simulink model "online_hardware_backstepping_controller"  (R2020b)
settings: Solver=FixedStepAuto  StartTime=0.0  StopTime=120  FixedStep=0.01  RelTol=1e-3  EnableMultiTasking=on
libraries: simulink x4, arduinolib x4, arduinosensorlib x1
settings Model: SILPILModeSetting=veronly  ExtModeTrigDuration=2  Creator=Boreth  LastModifiedBy=ONLY-GOD
settings OptimizationCC: EnhancedBackFolding=on  PassReuseOutputArgsAs=Individual arguments  MaxStackSize=64  OptimizeBlockOrder=speed  DifferentSizesBufferReuse=on  EfficientTunableParamExpr=on
settings DebuggingCC: InheritedTsInSrcMsg=none  ParameterTunabilityLossMsg=error  ArithmeticOperatorsInVariantConditions=warning
settings HardwareCC: ProdBitPerPointer=32  ProdBitPerSizeT=32  ProdBitPerPtrDiffT=32  ProdLargestAtomicInteger=Long  ProdLargestAtomicFloat=Double  ProdWordSize=32  ProdHWDeviceType=ARM Compatible->ARM Cortex
settings SFSimCC: MATLABDynamicMemAlloc=off  CustomCodeUndefinedFunction=UseInterfaceOnly
settings RTWCC: Description=Embedded Coder  SystemTargetFile=ert.tlc  HardwareBoard=Arduino Due  TemplateMakefile=ert_default_tmf  GenerateReport=on  Toolchain=Arduino ARM  BuildConfiguration=Faster Runs  IncludeHyperlinkInReport=on  LaunchReport=on  GenerateTraceInfo=on  GenerateTraceReport=on  GenerateTraceReportSl=on  GenerateTraceReportSf=on  GenerateTraceReportEml=on
settings CodeAppCC: ForceParamTrailComments=on  IgnoreCustomStorageClasses=off  OperatorAnnotations=on  SimulinkDataObjDesc=on  SFDataObjDesc=on  InsertBlockDesc=on
settings ERTTargetCC: SupportContinuousTime=on  SupportVariableSizeSignals=on  ExtModeStaticAllocSize=24576

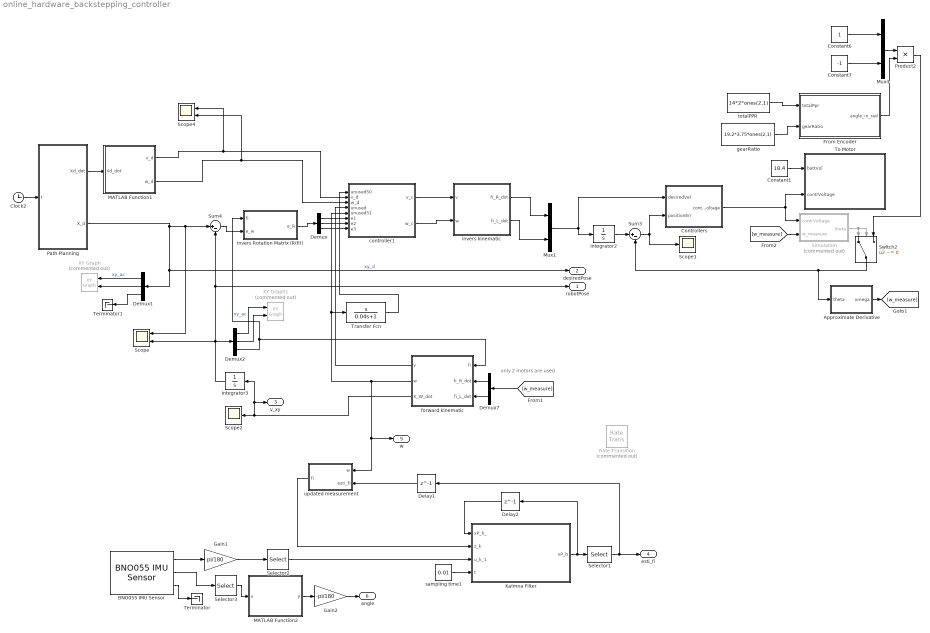
== system online_hardware_backstepping_controller ==
  note: only 2 motors are used
  Approximate Derivative : Subsystem
  BNO055 IMU Sensor : arduinosensorlib/BNO055 IMU Sensor  SlaveAddress=0x28  OperationMode=Fusion  Accel=off  AngularRate=on  MagField=off  EulerAngles=on  Quat=off  LinearAccel=off  GravityVector=off  AccelRange=4G  AccelBW=62.5 Hz  GyroRange=2000 dps  GyroBW=32 Hz  MagODR=10 Hz  SampleTime=0.01  blockPlatform=ARDUINO
      settings: SourceProductBaseCode=ARDUINO
  Clock2 : Clock
  Constant1 : Constant  Value=18.4
  Constant6 : Constant
  Constant7 : Constant  Value=-1
  Controllers : Subsystem
  Delay1 : Delay  DelayLength=1  InitialCondition=0
  Delay2 : Delay  DelayLength=1  InitialCondition=[0;0]
  Demux : Demux  Outputs=3
  Demux1 : Demux  Outputs=3
  Demux2 : Demux  Outputs=3
  Demux7 : Demux  Outputs=2
  From Encoder : Subsystem
  Gain1 : Gain  Gain=pi/180
  Gain2 : Gain  Gain=-pi/180
  Integrator2 : Integrator  InitialCondition=[0; 0]
  Integrator3 : Integrator  InitialCondition=[1.5;1;0]
  Kalmna Filter : MATLAB Function  TreatAsAtomicUnit=on
  MATLAB Function1 : MATLAB Function  TreatAsAtomicUnit=on
  MATLAB Function2 : MATLAB Function  TreatAsAtomicUnit=on
  Mux1 : Mux  Inputs=2
  Mux4 : Mux  Inputs=2
  Path Planning : MATLAB Function  TreatAsAtomicUnit=on
  Product2 : Product
  Rate Transition : RateTransition  Commented=on
  Scope : Scope  NumInputPorts=2
  Scope1 : Scope
  Scope2 : Scope
  Scope4 : Scope  NumInputPorts=2
  Selector1 : Selector  InputPortWidth=2  IndexOptions=Index vector (dialog)  Indices=1  OutputSizes=1
  Selector2 : Selector  InputPortWidth=3  IndexOptions=Index vector (dialog)  Indices=3  OutputSizes=1
  Selector3 : Selector  InputPortWidth=3  IndexOptions=Index vector (dialog)  Indices=1  OutputSizes=1
  Simulation : Subsystem  Commented=on
  Sum3 : Sum  Inputs=|+-
  Sum4 : Sum  Inputs=|+-
  Switch2 : Switch  Criteria=u2 ~= 0
  Terminator : Terminator
  Terminator1 : Terminator
  To Motor : Subsystem
  Transfer Fcn : TransferFcn  Numerator=[1 0]  Denominator=[0.04 1]
  XY Graph : simulink/Sinks/XY Graph  Commented=on  xmin=-5  xmax=5  ymin=-5  ymax=5  st=-1
  XY Graph1 : simulink/Sinks/XY Graph  Commented=on  xmin=-5  xmax=5  ymin=-5  ymax=5  st=-1
  controller1 : MATLAB Function  TreatAsAtomicUnit=on
  forward kinematic : MATLAB Function  TreatAsAtomicUnit=on
  gearRatio : Constant  Value=19.2*3.75*ones(2,1)
  invers Rotation Matrix (R(fi)) : MATLAB Function  TreatAsAtomicUnit=on
  invers kinematic : MATLAB Function  TreatAsAtomicUnit=on
  sampling time1 : Constant  Value=0.01
  totalPPR : Constant  Value=14*2*ones(2,1)
  updated measurement : MATLAB Function  TreatAsAtomicUnit=on
  robotPose : Outport
  desiredPose : Outport  Port=2
  v_xy : Outport  Port=3
  esti_fi : Outport  Port=4
  w : Outport  Port=5
  angle : Outport  Port=6
  wires:
  Approximate Derivative/1(omega) -> [w_measure]
  Controllers/1(contrVoltage) -> To Motor/2(contrVoltage), Simulation/1(contrVoltage)
  [w_measure] -> Simulation/2(w_measure)
  Mux1/1 -> Controllers/1(desiredVel), Integrator2/1
  Integrator2/1 -> Sum3/1
  Simulation/1(theta) -> Switch2/2, Switch2/1
  From Encoder/1(angle_in_rad) -> Product2/2
  Sum3/1 -> Scope1/1, Controllers/2(positionErr)
  Mux4/1 -> Product2/1
  Switch2/1 -> Approximate Derivative/1(theta), Sum3/2
  Constant7/1 -> Mux4/2
  Constant6/1 -> Mux4/1
  Product2/1 -> Switch2/3
  Path Planning/2(X_d) -> Demux1/1, desiredPose/1, Scope/1, Sum4/1  "xy_d"
  Demux2/3 -> forward kinematic/1(fi), invers Rotation Matrix (R(fi))/1(fi)
  Demux7/1 -> forward kinematic/2(fi_R_dot)
  Demux2/1 -> XY Graph1/1  "xy_ac"
  invers kinematic/1(fi_R_dot) -> Mux1/1
  Demux7/2 -> forward kinematic/3(fi_L_dot)
  Integrator3/1 -> Sum4/2, robotPose/1, Demux2/1, Scope/2
  invers kinematic/2(fi_L_dot) -> Mux1/2
  [w_measure] -> Demux7/1
  totalPPR/1 -> From Encoder/1(totalPpr)
  gearRatio/1 -> From Encoder/2(gearRatio)
  Constant1/1 -> To Motor/1(battVol)
  controller1/1(v_c) -> invers kinematic/1(v)
  controller1/2(w_c) -> invers kinematic/2(w)
  forward kinematic/1(v) -> controller1/4(unused)
  forward kinematic/2(w) -> w/1, updated measurement/1(w), controller1/5(unused51), Transfer Fcn/1
  Transfer Fcn/1 -> controller1/1(unused50)
  Clock2/1 -> Path Planning/1(t)
  Demux1/2 -> XY Graph/2
  Demux1/1 -> XY Graph/1  "xy_ac"
  Demux1/3 -> Terminator1/1
  Demux2/2 -> XY Graph1/2
  Demux/1 -> controller1/6(e1)
  Demux/2 -> controller1/7(e2)
  Demux/3 -> controller1/8(e3)
  Path Planning/1(Xd_dot) -> MATLAB Function1/1(Xd_dot)
  invers Rotation Matrix (R(fi))/1(e_R) -> Demux/1
  Sum4/1 -> invers Rotation Matrix (R(fi))/2(e_w)
  MATLAB Function1/2(w_d) -> Scope4/2, controller1/3(w_d)
  MATLAB Function1/1(v_d) -> Scope4/1, controller1/2(v_d)
  forward kinematic/3(X_W_dot) -> v_xy/1, Integrator3/1, Scope2/1
  BNO055 IMU Sensor/3 -> Terminator/1
  Gain2/1 -> angle/1
  Gain1/1 -> Selector2/1
  Selector3/1 -> MATLAB Function2/1(u)
  MATLAB Function2/1(y) -> Gain2/1
  Selector1/1 -> Delay1/1, esti_fi/1
  Delay2/1 -> Kalmna Filter/1(xP_h_)
  sampling time1/1 -> Kalmna Filter/4(t)
  BNO055 IMU Sensor/2 -> Selector3/1
  BNO055 IMU Sensor/1 -> Gain1/1
  Selector2/1 -> Kalmna Filter/3(u_k_1)
  Kalmna Filter/1(xP_h) -> Delay2/1, Selector1/1
  updated measurement/1(fi) -> Kalmna Filter/2(z_k)
  Delay1/1 -> updated measurement/2(esti_fi)

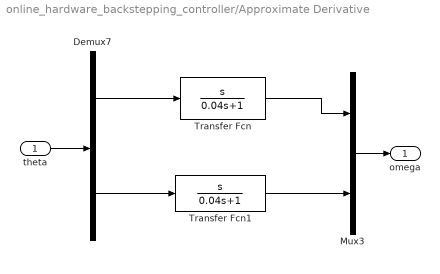
== system online_hardware_backstepping_controller/Approximate Derivative ==
  theta : Inport
  Demux7 : Demux  Outputs=2
  Mux3 : Mux  Inputs=2
  Transfer Fcn : TransferFcn  Numerator=[1 0]  Denominator=[0.04 1]
  Transfer Fcn1 : TransferFcn  Numerator=[1 0]  Denominator=[0.04 1]
  omega : Outport
  wires:
  Transfer Fcn1/1 -> Mux3/2
  Transfer Fcn/1 -> Mux3/1
  Mux3/1 -> omega/1
  Demux7/1 -> Transfer Fcn/1
  Demux7/2 -> Transfer Fcn1/1
  theta/1 -> Demux7/1

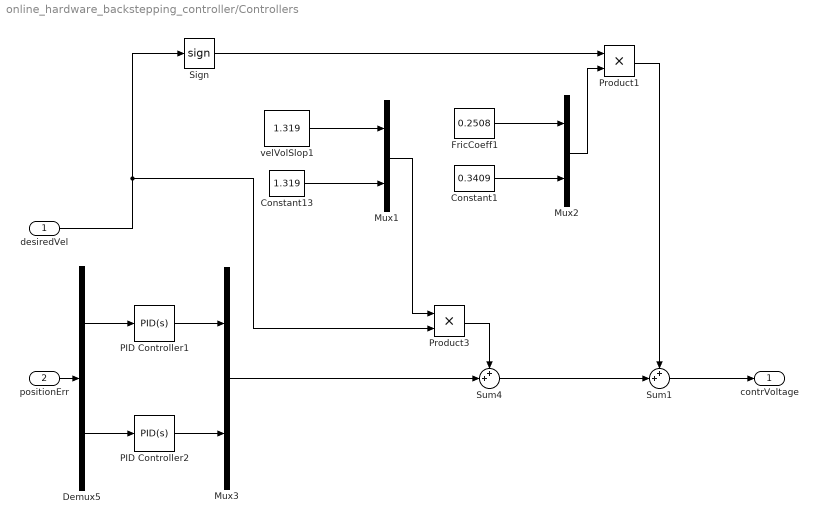
== system online_hardware_backstepping_controller/Controllers ==
  desiredVel : Inport
  positionErr : Inport  Port=2
  Constant1 : Constant  Value=0.3409
  Constant13 : Constant  Value=1.319
  Demux5 : Demux  Outputs=2
  FricCoeff1 : Constant  Value=0.2508
  Mux1 : Mux  Inputs=2
  Mux2 : Mux  Inputs=2
  Mux3 : Mux  Inputs=2
  "PID Controller1 " : simulink/Continuous/PID Controller  Controller=PID  Form=Parallel  TimeDomain=Continuous-time  SampleTime=-1  IntegratorMethod=Forward Euler  FilterMethod=Forward Euler  ControllerParametersSource=internal  P=60  I=0  D=3  UseFilter=on  N=50  TunerSelectOption=Transfer Function Based (PID Tuner App)  InitialConditionSource=internal  InitialConditionForIntegrator=0  InitialConditionForFilter=0  DifferentiatorICPrevScaledInput=0  ExternalReset=none  TrackingMode=off  Kt=1  LimitOutput=off  UpperSaturationLimit=inf  LowerSaturationLimit=-inf  LinearizeAsGain=on  AntiWindupMode=none  Kb=1  POutMin=[]  POutMax=[]  IOutMin=[]  IOutMax=[]  DOutMin=[]  DOutMax=[]  NOutMin=[]  NOutMax=[]  SumOutMin=[]  SumOutMax=[]  SaturationOutMin=[]  SaturationOutMax=[]  PParamMin=[]  PParamMax=[]  IParamMin=[]  IParamMax=[]  DParamMin=[]  DParamMax=[]  NParamMin=[]  NParamMax=[]  KbParamMin=[]  KbParamMax=[]  KtParamMin=[]  KtParamMax=[]  KbOutMin=[]  KbOutMax=[]  KtOutMin=[]  KtOutMax=[]  IntegratorOutMin=[]  IntegratorOutMax=[]  FilterOutMin=[]  FilterOutMax=[]  SumI1OutMin=[]  SumI1OutMax=[]  SumI2OutMin=[]  SumI2OutMax=[]  SumI3OutMin=[]  SumI3OutMax=[]  SumI4OutMin=[]  SumI4OutMax=[]  SumDOutMin=[]  SumDOutMax=[]  DifferentiatorOutMin=[]  DifferentiatorOutMax=[]  FilterDiffOutCoefMin=[]  FilterDiffOutCoefMax=[]  ReciprocalOutMin=[]  ReciprocalOutMax=[]  SumDenOutMin=[]  SumDenOutMax=[]  SumNumOutMin=[]  SumNumOutMax=[]  DivideOutMin=[]  DivideOutMax=[]  IntegratorContinuousStateAttributes=''  IntegratorStateMustResolveToSignalObject=off  IntegratorRTWStateStorageClass=Auto  FilterContinuousStateAttributes=''  FilterStateMustResolveToSignalObject=off  FilterRTWStateStorageClass=Auto  ParallelPVariant=InternalParameters  IdealPVariant=Disabled  IVariant=InternalParameters  DVariant=InternalParameters  IntegratorVariant=Continuous  SatVariant=Disabled  AWVariant=Passthrough  PCopyVariant=Disabled  TRVariant=Disabled  FdbkBlocksVariant=Forward  IdealPFdbkVariant=Disabled  SatFdbkVariant=Disabled  DerivativeFilterVariant=ContFilter  NVariant=InternalParameters  NCopyVariant=Disabled  FilterICVariant=InternalICsFilter  IntegratorICVariant=InternalICs  ExternalResetVariant=Disabled  TRSumVariant=Passthrough  SumFdbkVariant=Disabled  SumVariant=Sum_PID
  PID Controller2 : simulink/Continuous/PID Controller  Controller=PID  Form=Parallel  TimeDomain=Continuous-time  SampleTime=-1  IntegratorMethod=Forward Euler  FilterMethod=Forward Euler  ControllerParametersSource=internal  P=60  I=0  D=3  UseFilter=on  N=100  TunerSelectOption=Transfer Function Based (PID Tuner App)  InitialConditionSource=internal  InitialConditionForIntegrator=0  InitialConditionForFilter=0  DifferentiatorICPrevScaledInput=0  ExternalReset=none  TrackingMode=off  Kt=1  LimitOutput=off  UpperSaturationLimit=inf  LowerSaturationLimit=-inf  LinearizeAsGain=on  AntiWindupMode=none  Kb=1  POutMin=[]  POutMax=[]  IOutMin=[]  IOutMax=[]  DOutMin=[]  DOutMax=[]  NOutMin=[]  NOutMax=[]  SumOutMin=[]  SumOutMax=[]  SaturationOutMin=[]  SaturationOutMax=[]  PParamMin=[]  PParamMax=[]  IParamMin=[]  IParamMax=[]  DParamMin=[]  DParamMax=[]  NParamMin=[]  NParamMax=[]  KbParamMin=[]  KbParamMax=[]  KtParamMin=[]  KtParamMax=[]  KbOutMin=[]  KbOutMax=[]  KtOutMin=[]  KtOutMax=[]  IntegratorOutMin=[]  IntegratorOutMax=[]  FilterOutMin=[]  FilterOutMax=[]  SumI1OutMin=[]  SumI1OutMax=[]  SumI2OutMin=[]  SumI2OutMax=[]  SumI3OutMin=[]  SumI3OutMax=[]  SumI4OutMin=[]  SumI4OutMax=[]  SumDOutMin=[]  SumDOutMax=[]  DifferentiatorOutMin=[]  DifferentiatorOutMax=[]  FilterDiffOutCoefMin=[]  FilterDiffOutCoefMax=[]  ReciprocalOutMin=[]  ReciprocalOutMax=[]  SumDenOutMin=[]  SumDenOutMax=[]  SumNumOutMin=[]  SumNumOutMax=[]  DivideOutMin=[]  DivideOutMax=[]  IntegratorContinuousStateAttributes=''  IntegratorStateMustResolveToSignalObject=off  IntegratorRTWStateStorageClass=Auto  FilterContinuousStateAttributes=''  FilterStateMustResolveToSignalObject=off  FilterRTWStateStorageClass=Auto  ParallelPVariant=InternalParameters  IdealPVariant=Disabled  IVariant=InternalParameters  DVariant=InternalParameters  IntegratorVariant=Continuous  SatVariant=Disabled  AWVariant=Passthrough  PCopyVariant=Disabled  TRVariant=Disabled  FdbkBlocksVariant=Forward  IdealPFdbkVariant=Disabled  SatFdbkVariant=Disabled  DerivativeFilterVariant=ContFilter  NVariant=InternalParameters  NCopyVariant=Disabled  FilterICVariant=InternalICsFilter  IntegratorICVariant=InternalICs  ExternalResetVariant=Disabled  TRSumVariant=Passthrough  SumFdbkVariant=Disabled  SumVariant=Sum_PID
  Product1 : Product
  Product3 : Product
  Sign : Signum
  Sum1 : Sum  Inputs=++|
  Sum4 : Sum  Inputs=++|
  velVolSlop1 : Constant  Value=1.319
  contrVoltage : Outport
  wires:
  PID Controller2/1 -> Mux3/2
  Demux5/1 -> "PID Controller1 "/1
  "PID Controller1 "/1 -> Mux3/1
  positionErr/1 -> Demux5/1
  Demux5/2 -> PID Controller2/1
  Constant13/1 -> Mux1/2
  velVolSlop1/1 -> Mux1/1
  Mux1/1 -> Product3/1
  Sum1/1 -> contrVoltage/1
  Mux3/1 -> Sum4/2
  desiredVel/1 -> Sign/1, Product3/2
  Sum4/1 -> Sum1/2
  FricCoeff1/1 -> Mux2/1
  Constant1/1 -> Mux2/2
  Sign/1 -> Product1/1
  Mux2/1 -> Product1/2
  Product1/1 -> Sum1/1
  Product3/1 -> Sum4/1

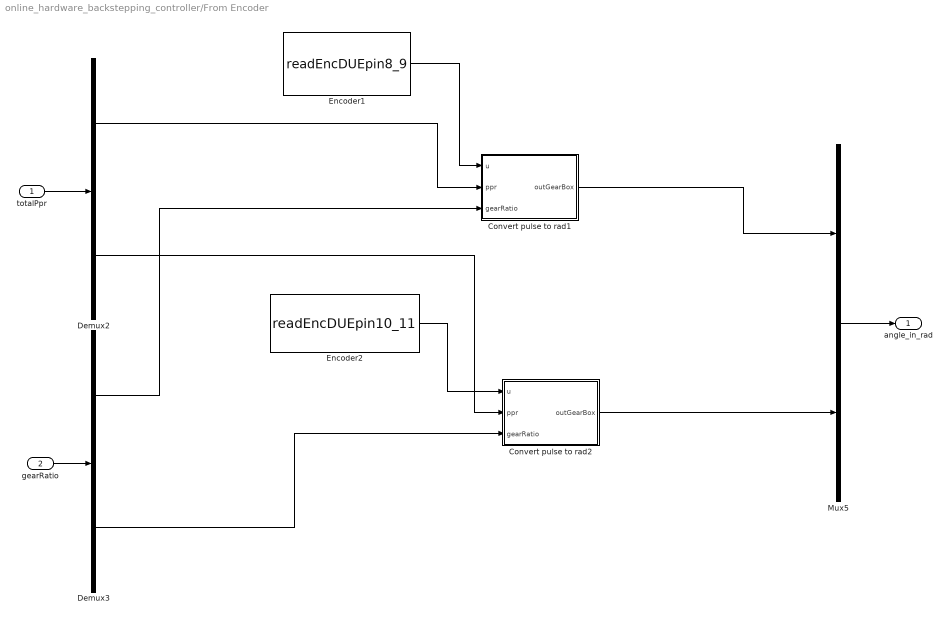
== system online_hardware_backstepping_controller/From Encoder ==
  totalPpr : Inport
  gearRatio : Inport  Port=2
  Convert pulse to rad1 : MATLAB Function  TreatAsAtomicUnit=on
  Convert pulse to rad2 : MATLAB Function  TreatAsAtomicUnit=on
  Demux2 : Demux  Outputs=2
  Demux3 : Demux  Outputs=2
  Encoder1 : S-Function  InitFcn=try, set_param(gcb,'FunctionName','readEncDUEpin8_9'), end  FunctionName=readEncDUEpin8_9  SFunctionModules=readEncDUEpin8_9_wrapper  SFunctionDeploymentMode=off  EnableBusSupport=off  mask(S-Function Builder){}
      mask help: Simulink:masks:SFunctionBuilder_MD
      mask init:
      | val = [[.9  0.75 0.75 1 1 .9 .9 1]',[1 1 0.75 0.75 .9 .9 1 .9]'];try , sys = get_param(gcb,'SfunBuilderFcnName');if isempty(sys), sys = get_param(gcb,'FunctionName'); end,catch, sys = get_param(gcb,'FunctionName'); end
      settings: CopyFcn=set_param(gcbh,'LinkStatus','none')  PreSaveFcn=try, set_param(gcb,'FunctionName','readEncDUEpin8_9'), end  OpenFcn=sfunctionwizard(gcbh)
      mask Display: plot(val(:,1),val(:,2)),disp(sys), port_label('output',1,'count')
  Encoder2 : S-Function  InitFcn=try, set_param(gcb,'FunctionName','readEncDUEpin10_11'), end  FunctionName=readEncDUEpin10_11  SFunctionModules=readEncDUEpin10_11_wrapper  SFunctionDeploymentMode=off  EnableBusSupport=off  mask(S-Function Builder){}
      mask help: Simulink:masks:SFunctionBuilder_MD
      mask init: same as online_hardware_backstepping_controller/From Encoder/Encoder1
      settings: CopyFcn=set_param(gcbh,'LinkStatus','none')  PreSaveFcn=try, set_param(gcb,'FunctionName','readEncDUEpin10_11'), end  OpenFcn=sfunctionwizard(gcbh)
      mask Display: plot(val(:,1),val(:,2)),disp(sys), port_label('output',1,'countt')
  Mux5 : Mux  Inputs=2
  angle_in_rad : Outport
  wires:
  Demux3/1 -> Convert pulse to rad1/3(gearRatio)
  Mux5/1 -> angle_in_rad/1
  Demux2/2 -> Convert pulse to rad2/2(ppr)
  gearRatio/1 -> Demux3/1
  Encoder2/1 -> Convert pulse to rad2/1(u)
  Demux2/1 -> Convert pulse to rad1/2(ppr)
  Convert pulse to rad1/1(outGearBox) -> Mux5/1
  Demux3/2 -> Convert pulse to rad2/3(gearRatio)
  Convert pulse to rad2/1(outGearBox) -> Mux5/2
  totalPpr/1 -> Demux2/1
  Encoder1/1 -> Convert pulse to rad1/1(u)

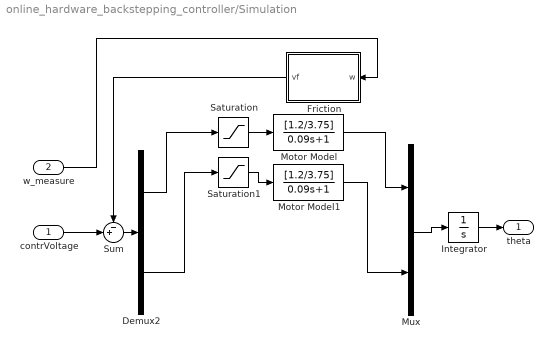
== system online_hardware_backstepping_controller/Simulation ==
  contrVoltage : Inport
  w_measure : Inport  Port=2
  Demux2 : Demux  Outputs=2
  Friction : MATLAB Function  TreatAsAtomicUnit=on
  Integrator : Integrator  InitialCondition=[0 0]
  Motor Model : TransferFcn  Numerator=[1.2/3.75]  Denominator=[0.09 1]
  Motor Model1 : TransferFcn  Numerator=[1.2/3.75]  Denominator=[0.09 1]
  Mux : Mux  Inputs=2
  Saturation : Saturate  UpperLimit=19  LowerLimit=-19
  Saturation1 : Saturate  UpperLimit=19  LowerLimit=-19
  Sum : Sum  Inputs=-+|
  theta : Outport
  wires:
  contrVoltage/1 -> Sum/2
  Demux2/1 -> Saturation/1
  Demux2/2 -> Saturation1/1
  Mux/1 -> Integrator/1
  Friction/1(vf) -> Sum/1
  Sum/1 -> Demux2/1
  w_measure/1 -> Friction/1(w)
  Integrator/1 -> theta/1
  Motor Model/1 -> Mux/1
  Motor Model1/1 -> Mux/2
  Saturation/1 -> Motor Model/1
  Saturation1/1 -> Motor Model1/1

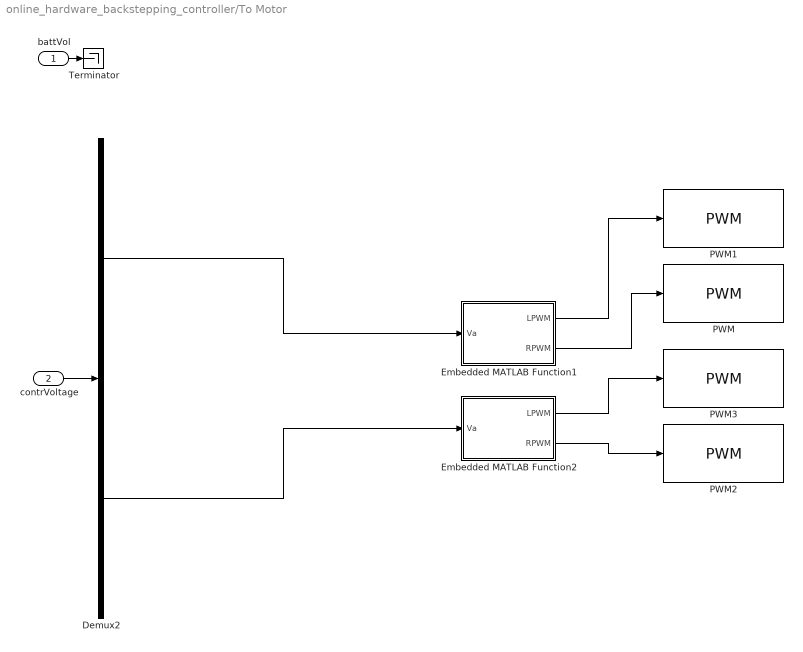
== system online_hardware_backstepping_controller/To Motor ==
  battVol : Inport
  contrVoltage : Inport  Port=2
  Demux2 : Demux  Outputs=2
  Embedded MATLAB Function1 : MATLAB Function  TreatAsAtomicUnit=on
  Embedded MATLAB Function2 : MATLAB Function  TreatAsAtomicUnit=on
  PWM : arduinolib/PWM  pinNumber=6  frequencyType=Default  desiredFrequency=490.2  achievableFrequency=490.2
  PWM1 : arduinolib/PWM  pinNumber=7  frequencyType=Default  desiredFrequency=490.2  achievableFrequency=490.2
  PWM2 : arduinolib/PWM  pinNumber=4  frequencyType=Default  desiredFrequency=490.2  achievableFrequency=490.2
  PWM3 : arduinolib/PWM  pinNumber=5  frequencyType=Default  desiredFrequency=490.2  achievableFrequency=490.2
  Terminator : Terminator
  wires:
  contrVoltage/1 -> Demux2/1
  Embedded MATLAB Function1/1(LPWM) -> PWM1/1
  Embedded MATLAB Function1/2(RPWM) -> PWM/1
  Embedded MATLAB Function2/1(LPWM) -> PWM3/1
  Embedded MATLAB Function2/2(RPWM) -> PWM2/1
  battVol/1 -> Terminator/1
  Demux2/1 -> Embedded MATLAB Function1/1(Va)
  Demux2/2 -> Embedded MATLAB Function2/1(Va)

== matlab function online_hardware_backstepping_controller/To Motor/Embedded MATLAB Function2 ==
  data: Va input; LPWM output; RPWM output
function [LPWM,RPWM] = fcn(Va)

Vmax = 18.4; % supply voltage is Vmax = 18.4v
PWM = abs(Va)*255/Vmax;
if PWM > 255
    PWM = 255;
end
if Va>=0
    LPWM = PWM;
    RPWM = 0;
else
    LPWM = 0;
    RPWM = PWM;
end

== matlab function online_hardware_backstepping_controller/forward kinematic ==
  data: v output; w output; fi input; fi_R_dot input; X_W_dot output; fi_L_dot input
function [v, w, X_W_dot] = M_inv(fi,fi_R_dot, fi_L_dot)
r = 0.07;      %wheel radius
b = 0.22; 

v = r*[0.5 0.5]*[fi_R_dot; fi_L_dot];
w = r*[0.5/b -0.5/b]*[fi_R_dot; fi_L_dot];
X_W_dot = [cos(fi) 0;sin(fi) 0; 0 1]*[v; w];

== matlab function online_hardware_backstepping_controller/invers Rotation Matrix (R(fi)) ==
  data: fi input; e_R output; e_w input
function e_R = fcn(fi,e_w)
%#codegen

R = [cos(fi), sin(fi), 0; -sin(fi), cos(fi), 0; 0, 0, 1];
e_R = R*e_w;

== matlab function online_hardware_backstepping_controller/invers kinematic ==
  data: v input; fi_R_dot output; w input; fi_L_dot output
function [fi_R_dot, fi_L_dot] = M_inv(v, w)
r = 0.07;      %wheel radius
b = 0.22; 
fi_R_dot = (v + w*b)/r;
fi_L_dot = (v - w*b)/r;

== matlab function online_hardware_backstepping_controller/Kalmna Filter ==
  data: xP_h_ input; xP_h output; z_k input; u_k_1 input; t input
function xP_h = fcn(xP_h_, z_k, u_k_1, t)

A = 1;

H = 1;

B = t;
R = 1e-3;
Q = 1e-1;

x = xP_h_(1);
P = xP_h_(2);
%P = reshape(P,5,5);
x = A*x + B*u_k_1;
P = A*P*A' + Q;
z = H*x;
P_xz = P*H';
P_zz = H*P*H' + R;
x = x + (P_xz/P_zz)*(z_k - z);
P = P - (P_xz/P_zz)*P_xz';

xP_h = [x;P];

== matlab function online_hardware_backstepping_controller/MATLAB Function2 ==
  data: u input; y output
function y = detectjump(u)
persistent detect_jump u_1
if isempty(detect_jump)
    detect_jump = 0; u_1 = 0;
end

if u - u_1 > 355
    detect_jump = detect_jump -1;
end

if u - u_1 < -355
    detect_jump = detect_jump +1;
end
y = u +detect_jump*360;

u_1 = u;

== matlab function online_hardware_backstepping_controller/updated measurement ==
  data: w input; fi output; esti_fi input
function fi = fcn(w, esti_fi)

d_fi = 0.01*w; %sampling time = 0.01
fi = d_fi + esti_fi;

== matlab function online_hardware_backstepping_controller/Path Planning ==
  data: Xd_dot output; t input; X_d output
function [Xd_dot,X_d ]=  fcn(t)
%#codegen

%Straght-line Trajectroy Tracking
% v=2;
% x_d= -0.5 + v*t;
% y_d= 0.5 +v*t;
% theta_d=pi/2;
% X_d=[x_d;y_d;theta_d];

% xd_dot=v;
% yd_dot=v;
% thetad_dot=0;
%Xd_dot=[xd_dot;yd_dot;thetad_dot];

% Circular Trajectory Tracking
% w0=pi/2;
% wr=0.2;
% r=3;
% x_d=r*cos(w0+wr*t);
% y_d=r*sin(w0+wr*t);
% theta_d=pi/2;

r = 1.5;
wr = 0.1;
x_d= r*cos(wr*t);
y_d= 1 - r*sin(wr*t);
theta_d=0;

X_d=[x_d;y_d;theta_d];

xd_dot=-r*wr*sin(wr*t);
yd_dot=r*wr*cos(wr*t);
thetad_dot=0;

Xd_dot=[xd_dot;yd_dot;thetad_dot];

== matlab function online_hardware_backstepping_controller/From Encoder/Convert pulse to rad1 ==
  settings: updateMethod=DISCRETE
  data: u input; ppr input; gearRatio input; outGearBox output
function outGearBox = fcn(u,ppr,gearRatio)

persistent counter_num over_flag
if(isempty(counter_num)), counter_num = 0;end
if(isempty(over_flag)), over_flag = 0;end
pulse2radian = 2*pi/ppr; % 1 pulse = ?? radian

if(double(u) - counter_num > 40000), over_flag = over_flag-1;
elseif(double(u) - counter_num < -40000), over_flag = over_flag+1;
end

inGearBox = (double(u)+over_flag*(2^32 -1))*pulse2radian; 
outGearBox = inGearBox/gearRatio;
counter_num = double(u) ;

== matlab function online_hardware_backstepping_controller/From Encoder/Convert pulse to rad2 ==
  settings: updateMethod=DISCRETE
  data: u input; ppr input; gearRatio input; outGearBox output
function outGearBox = fcn(u,ppr,gearRatio)

persistent counter_num over_flag
if(isempty(counter_num)), counter_num = 0;end
if(isempty(over_flag)), over_flag = 0;end
pulse2radian = 2*pi/ppr; % 1 pulse = ?? radian

if(double(u) - counter_num > 40000), over_flag = over_flag-1;
elseif(double(u) - counter_num < -40000), over_flag = over_flag+1;
end

inGearBox = (double(u)+over_flag*(2^32 -1))*pulse2radian; 
outGearBox = inGearBox/gearRatio;
counter_num = double(u) ;

== matlab function online_hardware_backstepping_controller/Simulation/Friction ==
  data: w input; vf output
function vf = fcn(w)

vf = 0.13*sigmoidFcn(w);
end

function y = sigmoidFcn(x)
y = 2./(1+exp(-15*x))-1; % element wise computing
end

== matlab function online_hardware_backstepping_controller/controller1 ==
  data: unused50 input; v_d input; w_d input; unused input; unused51 input; e1 input; v_c output; w_c output; e2 input; e3 input
function [v_c,w_c] =  fcn(~,v_d, w_d, ~, ~, e1, e2, e3)            


k1 = 1;
k2 = 20 ;
k3 = 1 ;
%lambda = 2 ;

% x_e_hat = e1 - k1*w*e2;
% v1 = w*e2 + v_d*cos(e3) - v - k1*w_dot*e2 + k1*w*(w*e1 - v_d*sin(e3));
% v_c = v1 - e2*w + k2*x_e_hat;
% w_c = w_d + lambda*e2*v_d*i + k3*lambda*e3;
%w_c = w_d +k3*lambda*e3;

v_c = k1*e1 + v_d*cos(e3);
w_c = w_d + k2*v_d*e2 + k3*v_d*sin(e3);

== matlab function online_hardware_backstepping_controller/MATLAB Function1 ==
  data: Xd_dot input; v_d output; w_d output
function [v_d, w_d] = fcn(Xd_dot)

v_d = sqrt(Xd_dot(1)^2 + Xd_dot(2)^2);
w_d = Xd_dot(3);

== matlab function online_hardware_backstepping_controller/To Motor/Embedded MATLAB Function1 ==
  data: Va input; LPWM output; RPWM output
function [LPWM,RPWM] = fcn(Va)

Vmax = 18.4; % supply voltage is Vmax = 18.4v
PWM = abs(Va)*255/Vmax;
if PWM > 255
    PWM = 255;
end
if Va>=0
    LPWM = PWM;
    RPWM = 0;
else
    LPWM = 0;
    RPWM = PWM;
end
